simulink subsystem "BTS"  (R2024a)
settings: Solver=VariableStepAuto  StartTime=0.0  StopTime=10.0  RelTol=1e-3
settings Model: Creator=nicol  LastModifiedBy=nicol

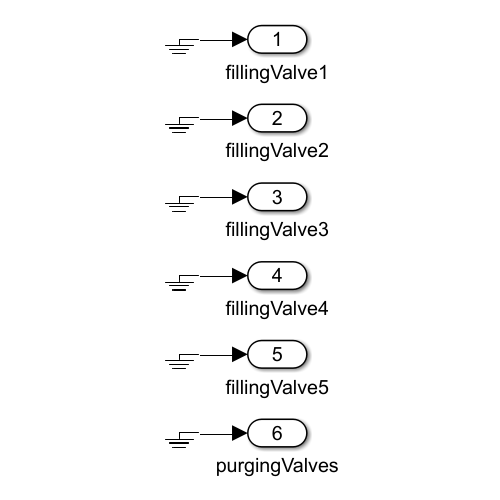
[thumbnail: Simulink's stored preview of the top-level diagram]
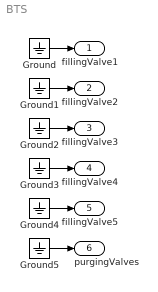
== system BTS ==
  Ground{,1..5} (6 alike) : Ground
  fillingValve1 : Outport
  fillingValve2 : Outport  Port=2
  fillingValve3 : Outport  Port=3
  fillingValve4 : Outport  Port=4
  fillingValve5 : Outport  Port=5
  purgingValves : Outport  Port=6
  wires:
  Ground/1 -> fillingValve1/1
  Ground1/1 -> fillingValve2/1
  Ground2/1 -> fillingValve3/1
  Ground3/1 -> fillingValve4/1
  Ground4/1 -> fillingValve5/1
  Ground5/1 -> purgingValves/1
